simulink model "CONTROL_TESTING"  (R2024a)
settings: Solver=VariableStepAuto  StartTime=0.0  StopTime=inf  RelTol=1e-3
values from neighbouring files (symbols this model uses):
  C = 0    [CONTROL_TESTING_VARIABLES.m]
  Direction_Pin = 0    [CONTROL_TESTING_VARIABLES.m]
  EN_Pin = 1    [CONTROL_TESTING_VARIABLES.m]
  FP_New_Max_Angle = 360    [CONTROL_TESTING_VARIABLES.m]
  FP_New_Max_Percent = 255    [CONTROL_TESTING_VARIABLES.m]
  FP_New_Min_Angle = 0    [CONTROL_TESTING_VARIABLES.m]
  FP_New_Min_Percent = 0    [CONTROL_TESTING_VARIABLES.m]
  FP_Old_Max = 5    [CONTROL_TESTING_VARIABLES.m]
  FP_Old_Min = 0    [CONTROL_TESTING_VARIABLES.m]
  TB_New_Max_Angle = 360    [CONTROL_TESTING_VARIABLES.m]
  TB_New_Max_Percent = 255    [CONTROL_TESTING_VARIABLES.m]
  TB_New_Min_Angle = 0    [CONTROL_TESTING_VARIABLES.m]
  TB_New_Min_Percent = 0    [CONTROL_TESTING_VARIABLES.m]
  TB_Old_Max = 5    [CONTROL_TESTING_VARIABLES.m]
  TB_Old_Min = 0    [CONTROL_TESTING_VARIABLES.m]
libraries: fl_lib x11, nesl_utility x9, arduinolib x4, ee_lib x3, sdl_lib x1
(part 1 of 2)
settings Model: Creator=Banana444  LastModifiedBy=Banana444

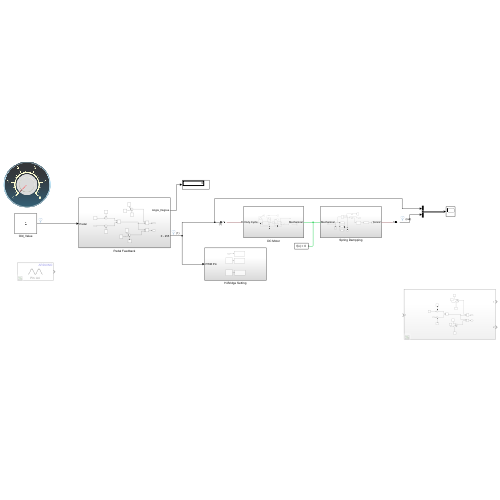
[thumbnail: Simulink's stored preview of the top-level diagram]
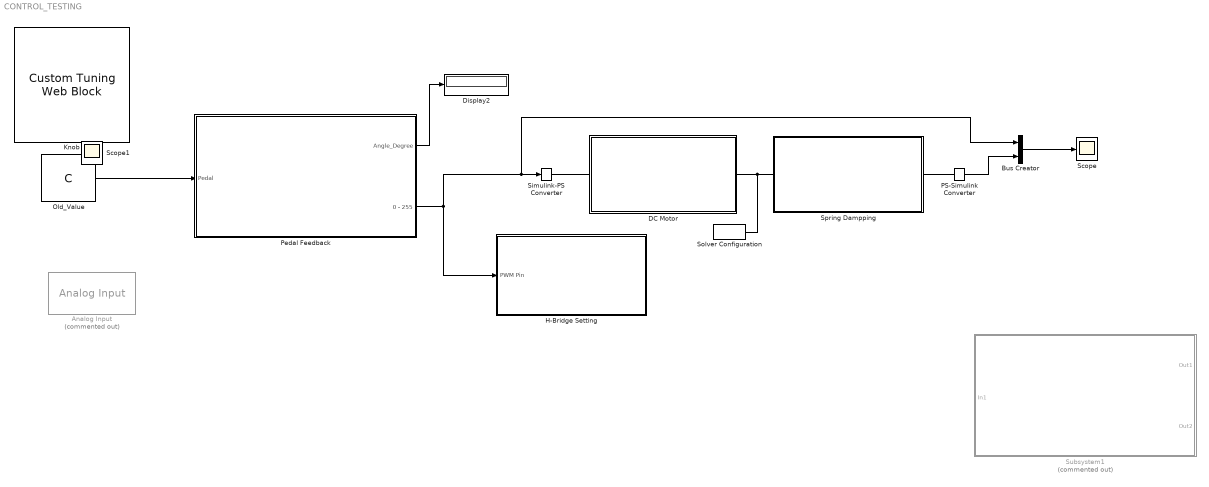
== system CONTROL_TESTING ==
  Analog Input : arduinolib/Analog Input  Commented=on  pinNumber=4  ReadResultsOnly=off  ConversionTriggerSource=Software  ExternalTriggerType=uint32( 0 )  OutputDataType=uint16  EnableConversionCompleteNotify=off  EnableOuputStatus=off  SampleTime=-1  blockPlatform=arduino
  Bus Creator : BusCreator  Inputs=2
  DC Motor : Subsystem
  Display2 : Display
  H-Bridge Setting : Subsystem
  Knob : CustomTuningWebBlock  LabelPosition=Hide  ShowInitialText=on  Configuration="{\"components\":[{\"name\":\"CircularScaleComponent\",\"settings\":{\"bounds\":{\"max\":5,\"min\":0,\"tickInterval\":\"auto\"},\"direction\":\"cw\",\"flipLimits\":0,\"innerRadius\":0.6636618227670849,\"internalTickHeightScaleFactor\":1,\"labelColor\":[255,255,200],\"labelFont\":{\"font\":\"Arial\",\"fontSize\":12},\"labelRadius\":0.79,\"labelTransparency\":1,\"minorTickHeightScaleFactor\":0.2,\"needleImage\":{\"size\":[150,150],\"src\":\"data:image\\/svg+xml;base64,PD94bWwgdmVyc2lvbj0iMS4wIiBlbmNvZGluZz0idXRmLTgiPz4NCjwhLS0gR2VuZXJhdG9yOiBBZG9iZSBJbGx1c3RyYXRvciAyNS4yLjMsIFNWRyBFeHBvcnQgUGx1Zy1JbiAuIFNWRyBWZXJzaW9uOiA2LjAwIEJ1aWxkIDApICAtLT4NCjxzdmcgdmVyc2lvbj0iMS4xIiBpZD0iTGF5ZXJfMSIgeG1sbnM9Imh0dHA6Ly93d3cudzMub3JnLzIwMDAvc3ZnIiB4bWxuczp4bGluaz0iaHR0cDovL3d3dy53My5vcmcvMTk5OS94bGluayIgeD0iMHB4IiB5PSIwcHgiDQoJIHZpZXdCb3g9IjAgMCAxNTIgMTUyIiBzdHlsZT0iZW5hYmxl ...(+37472 chars)\"},\"needleOffset\":[0,0],\"needleOrientation\":-45,\"needleRotation\":90,\"needleSize\":{\"height\":0.44,\"width\":0.44},\"outerRadius\":0.5053386200069245,\"position\":[0,0,1,1],\"referencePoint\":\"auto\",\"scaleAngle\":270,\"scaleAngleOffset\":135,\"scaleColors\":[],\"scaleColorsSize\":0.2,\"scaleDirection\":\"CW\",\"scalePosition\":[0,0,1,1],\"showLabels\":1,\"showMinorTicks\":1,\"showSpanLine\":true,\"showTicks\":1,\"tickColor\":[252,252,197],\"tickTransparency\":1,\"valueBarColor\":[0,114,189],\"valueBarPosition\":[0,0,1,1],\"valueBarSize\":0.2,\"valueBarTransparency\":1}},{\"name\":\"BackgroundImageComponent\",\"settings\":{\"image\":{\"size\":[385,373],\"src\":\"data:image\\/svg+xml;base64,PD94bWwgdmVyc2lvbj0iMS4wIiBlbmNvZGluZz0idXRmLTgiPz4NCjwhLS0gR2VuZXJhdG9yOiBBZG9iZSBJbGx1c3RyYXRvciAyNS4wLjAsIFNWRyBFeHBvcnQgUGx1Zy1JbiAuIFNWRyBWZXJzaW9uOiA2LjAwIEJ1aWxkIDApICAtLT4NCjxzdmcgdmVyc2lvbj0iMS4xIg0KCSBpZD0iTGF5ZXJfMl8xXyIgeG1sbnM6Y2M9Imh0dHA6Ly9jcmVhdGl2ZWNvbW1vbnMub3JnL25zIyIgeG1sbnM6ZGM9Imh0dHA6Ly9wdXJsLm9yZy9kYy9lbGVtZW50cy8xLjEvIiB4bWxuczppbmtzY2FwZT0iaHR0cDovL3d3dy5pbmtzY2FwZS5vcmcv ...(+4184 chars)\",\"srcOrientation\":\"horizontal\"},\"position\":[0,0,1,1],\"scaleMode\":\"0\"}},{\"name\":\"ForegroundImageComponent\",\"settings\":{\"image\":{\"size\":[0,0],\"src\":\"default\",\"srcOrientation\":[]},\"isForeground\":1,\"position\":[0,0,1,1],\"scaleMode\":\"0\"}}],\"settings\":{\"BindingType\":\"param\",\"aspectRatio\":1,\"backgroundColor\":[0,0,0,\"1\"],\"backgroundOffset\":1,\"backgroundOpacity\":1,\"direction\":\"cw\",\"fixedAspectRatio\":\"on\",\"flipLimits\":0,\"foregroundColor\":[252,252,196],\"orientation\":\"horizontal\",\"showBackgroundColor\":false,\"value\":0,\"version\":\"R2023a\"},\"type\":\"CircularGauge\"}"
  Old_Value : Constant  Value=C
  PS-Simulink Converter : nesl_utility/PS-Simulink Converter  PhysicalDomain=network_engine_domain  SubClassName=ps_output  LeftPortType=input  RightPortType=output  PseudoPeriodic=off  Frequencies=[]  VectorFormat=inherit  Unit=inherit  AffineConversion=off
  Pedal Feedback : Subsystem
  Scope : Scope
  Simulink-PS Converter : nesl_utility/Simulink-PS Converter  PhysicalDomain=network_engine_domain  SubClassName=ps_input  LeftPortType=input  RightPortType=output  PseudoPeriodic=off  Frequencies=[]  NoiseDistribution=none  NoiseParameters=[]  Unit=1  AffineConversion=off  FilteringAndDerivatives=provide  SimscapeFilterOrder=1  InputFilterTimeConstant=0.001  UdotUserProvided=0
  Solver Configuration : nesl_utility/Solver Configuration  PhysicalDomain=network_engine_domain  SubClassName=solver  LeftPortType=input  RightPortType=generic  Tones=[]  Harmonics=[]  SimulateNoise=off  Profile=off  UseLocalSampling=off  EnableSwitchedLinearOptims=on  FrequencyDomain=off  UseCCode=off  RelTol=0.001  AbsTol=1e-06  MinStep=1e-09  ToWorkspace=off  RevertToSquareIcSolve=off  NumHomotopyIterations=100  PhasorMode=off  PhasorModeNumHarmonics=1  ConsistencySolver=NEWTON_FTOL  IndexReductionMethod=DerivativeReplacement  DoDC=off  ResidualTolerance=1e-9  ConsistencyTolSource=GLOBAL  ConsistencyAbsTol=0.001  ConsistencyRelTol=0.001  ConsistencyTolFactor=0.001  UseLocalSolver=off  LocalSolverChoice=NE_BACKWARD_EULER_ADVANCER  ResolveIndetEquations=on  FunctionEvalNumThread=1  LocalSolverSampleTime=5e-6  DoFixedCost=off  MaxNonlinIter=4  MaxModeIter=2  ComputeImpulses=off  ImpulseIterations=2  LinearAlgebra=auto  LinearAlgebraNumThread=0  EquationFormulation=NE_TIME_EF  DelaysMemoryBudget=1024  AutomaticFiltering=on  FilteringTimeConstant=0.001  PartitionStorageMethod=AS_NEEDED  PartitionMemoryBudget=1024  PartitionMethod=FAST  MultibodyUseLocalSolver=off  MultibodyLocalSolverChoice=ODE1  MultibodyLocalSolverSampleTime=0.001
  Spring Dampping : Subsystem
  Subsystem1 : Subsystem  Commented=on
  Scope1 : Scope
  wires:
  Pedal Feedback/2(0 - 255) -> H-Bridge Setting/1(PWM Pin), Bus Creator/1, Simulink-PS Converter/1
  Pedal Feedback/1(Angle_Degree) -> Display2/1
  PS-Simulink Converter/1 -> Bus Creator/2
  Bus Creator/1 -> Scope/1
  Old_Value/1 -> Pedal Feedback/1(Pedal)
  connections:
  Simulink-PS Converter/RConn1 -- DC Motor/LConn1
  DC Motor/RConn1 -- Solver Configuration/RConn1 -- Spring Dampping/LConn1
  Spring Dampping/RConn1 -- PS-Simulink Converter/LConn1
